simulink model "ssc_transformer"  (R2016b)
settings: Solver=VariableStepAuto  StartTime=0.0  StopTime=1  MaxStep=5e-5  RelTol=1e-3  EnableMultiTasking=on
PreLoadFcn:
  | L1 = 0.75*2.54e-2;  % 0.75 inch
  | L2 = 1.5*2.54e-2 ;  % 1.5 inch
  | Area = L1*L1;
libraries: fl_lib x19, nesl_utility x7
CloseFcn:
  | try,close(h1_ssc_transformer),end
  | clear h1_ssc_transformer
  | clear simlog_ssc_transformer
Description:
  | Electrical Transformer
  | 
  | Copyright 2008-2016 The MathWorks, Inc.
settings Model: Creator=MathWorks  LastModifiedBy=SHAAD
settings DataIOCC: LimitDataPoints=on  SaveFormat=Array
settings OptimizationCC: LifeSpan=inf
settings DebuggingCC: SolverPrmCheckMsg=warning  AllowSymbolicDim=off  SFUnexpectedBacktrackingDiag=warning  SFNoUnconditionalDefaultTransitionDiag=warning  SFExecutionAtInitializationDiag=none
settings HardwareCC: ProdBitPerPointer=32  ProdBitPerSizeT=32  ProdBitPerPtrDiffT=32  ProdLargestAtomicFloat=None  ProdIntDivRoundTo=Undefined  ProdEndianess=Unspecified  ProdWordSize=32  ProdHWDeviceType=32-bit Generic
settings ModelReferenceCC: PropagateSignalLabelsOutOfModel=off
settings GRTTargetCC: TargetLangStandard=C89/C90 (ANSI)  GeneratePreprocessorConditionals=Disable all
settings ConfigComp: CovMetricSettings=dw  CovHtmlReporting=on  CovSaveCumulativeToWorkspaceVar=on  CovSaveSingleToWorkspaceVar=on  CovExternalEMLEnable=off  CovSFcnEnable=off
settings SimscapeCC: SimscapeLogType=all  SimscapeLogSimulationStatistics=on  SimscapeLogName=simlog_ssc_transformer  SimscapeLogDataHistory=30000

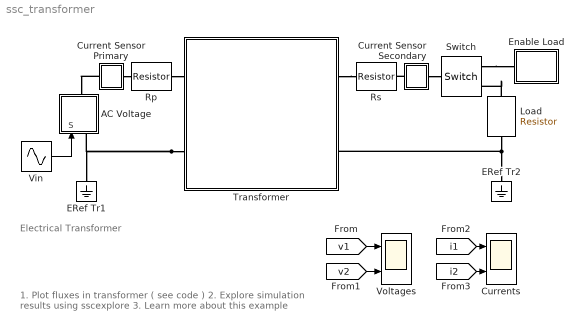
== system ssc_transformer ==
  note: 1. Plot fluxes in transformer ( see code )
      | 2. Explore simulation results using sscexplore
      | 3. Learn more about this example
  note: Electrical Transformer
  AC Voltage : Subsystem
  Current Sensor Primary : Subsystem
      mask Display: disp('vi1')
  Current Sensor Secondary : Subsystem
      mask Display: disp('vi2')
  Currents : Scope  NumInputPorts=2
  ERef Tr1 : fl_lib/Electrical/Electrical Elements/Electrical Reference
  ERef Tr2 : fl_lib/Electrical/Electrical Elements/Electrical Reference
  Enable Load : Subsystem
  Load : fl_lib/Electrical/Electrical Elements/Resistor  R=2.88 Ohm  i_specify=off  i_priority=High  i=0 A  v_specify=off  v_priority=High  v=0 V
  Rp : fl_lib/Electrical/Electrical Elements/Resistor  R=8.4683 Ohm  i_specify=off  i_priority=High  i=0 A  v_specify=off  v_priority=High  v=0 V
  Rs : fl_lib/Electrical/Electrical Elements/Resistor  R=8.4683/100 Ohm  i_specify=off  i_priority=High  i=0 A  v_specify=off  v_priority=High  v=0 V
  Switch : fl_lib/Electrical/Electrical Elements/Switch  R_closed=0.01 Ohm  G_open=1e-8 1/Ohm  Threshold=0  i_specify=off  i_priority=High  i=0 A  v_specify=off  v_priority=High  v=0 V
  Transformer : Subsystem  Tag=PublishSubsystem
      mask Display:
      | % Primary Coil
      | plot(cos(+pi/2:0.1:3*pi/2)*0.10-0.3,sin(+pi/2:0.1:3*pi/2)*0.10+0.4);
      | plot(cos(+pi/2:0.1:3*pi/2)*0.10-0.3,sin(+pi/2:0.1:3*pi/2)*0.10+0.2);
      | plot(cos(+pi/2:0.1:3*pi/2)*0.10-0.3,sin(+pi/2:0.1:3*pi/2)*0.10+0.0);
      | plot(cos(+pi/2:0.1:3*pi/2)*0.10-0.3,sin(+pi/2:0.1:3*pi/2)*0.10-0.2);
      | plot(cos(+pi/2:0.1:3*pi/2)*0.10-0.3,sin(+pi/2:0.1:3*pi/2)*0.10-0.4);
      | plot([-0.3 -0.3],[-0.6 -0.5]);plot([-0.3 -0.8],[-0.6 -0.6]);
      | plot([-0.3 -0.3],[+0.6 +0.5]);plot([-0.3 -0.8],[+0.6 +0.6]);
      | 
      | % Secondary Coil
      | plot(cos(-pi/2:0.1:pi/2)*0.10+0.3,sin(-pi/2:0.1:pi/2)*0.10+0.4);
      | plot(cos(-pi/2:0.1:pi/2)*0.10+0.3,sin(-pi/2:0.1:pi/2)*0.10+0.2);
      | plot(cos(-pi/2:0.1:pi/2)*0.10+0.3,sin(-pi/2:0.1:pi/2)*0.10+0.0);
      | plot(cos(-pi/2:0.1:pi/2)*0.10+0.3,sin(-pi/2:0.1:pi/2)*0.10-0.2);
      | plot(cos(-pi/2:0.1:pi/2)*0.10+0.3,sin(-pi/2:0.1:pi/2)*0.10-0.4);
      | plot([0.3 0.3],[-0.6 -0.5]);plot([0.3 0.8],[-0.6 -0.6]);
      | plot([0.3 0.3],[+0.6 +0.5]);plot([0.3 0.8],[+0.6 +0.6]);
      | 
      | % Plot points to set plot range
      | color('white');plot(1.1,1.1);plot(-1.1,-1.1)
      | color('black');
      | 
      | color('red')
      | port_label('LConn',1,'+1');
      | port_label('LConn',2,'-1');
      | port_label('RConn',1,'+2');
      | port_label('RConn',2,'-2');
      | color('black');
  Vin : Sin  Amplitude=120*sqrt(2)  Frequency=2*pi*60  Phase=pi/2  SampleTime=0
  Voltages : Scope  NumInputPorts=2
  wires:
  [v2] -> Voltages/2
  [v1] -> Voltages/1
  [i2] -> Currents/2
  [i1] -> Currents/1
  Vin/1 -> AC Voltage/1(S)
  connections:
  Current Sensor Secondary/RConn1 -- Switch/LConn1
  Load/RConn1 -- ERef Tr2/LConn1 -- Transformer/RConn2
  Load/LConn1 -- Switch/RConn2
  Rp/LConn1 -- Transformer/LConn1
  Transformer/RConn1 -- Rs/RConn1
  Current Sensor Secondary/LConn1 -- Rs/LConn1
  Transformer/LConn2 -- AC Voltage/LConn1 -- ERef Tr1/LConn1
  Current Sensor Primary/RConn1 -- Rp/RConn1
  Current Sensor Primary/LConn1 -- AC Voltage/RConn1
  Switch/RConn1 -- Enable Load/LConn1

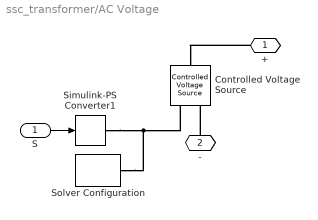
== system ssc_transformer/AC Voltage ==
  S : Inport
  Controlled Voltage Source : fl_lib/Electrical/Electrical Sources/Controlled Voltage Source
  Simulink-PS Converter1 : nesl_utility/Simulink-PS Converter  PhysicalDomain=network_engine_domain  SubClassName=ps_input  LeftPortType=input  RightPortType=output  PseudoPeriodic=off  Frequencies=[]  NoiseDistribution=none  NoiseParameters=[]  Unit=1  AffineConversion=off  InputFiltering=off  SimscapeFilterOrder=1  InputFilterTimeConstant=.001  UdotUserProvided=0
  Solver Configuration : nesl_utility/Solver Configuration  PhysicalDomain=network_engine_domain  SubClassName=solver  LeftPortType=input  RightPortType=generic  Accelerate=off  Tones=[]  Harmonics=[]  SimulateNoise=off  Profile=off  UseLocalSampling=off  EnableSwitchedLinearOptims=on  FrequencyDomain=off  UseCCode=off  RelTol=0.001  AbsTol=1e-06  MinStep=1e-09  ToWorkspace=off  RevertToSquareIcSolve=off  NumHomotopyIterations=100  PhasorMode=off  PhasorModeNumHarmonics=1  OverrideAbsTol=off  DoDC=off  ResidualTolerance=1e-9  UseLocalSolver=off  LocalSolverChoice=NE_BACKWARD_EULER_ADVANCER  LocalSolverSampleTime=.001  DoFixedCost=off  MaxNonlinIter=3  MaxModeIter=2  LinearAlgebra=Sparse  DelaysMemoryBudget=1024  AutomaticFiltering=on  FilteringTimeConstant=0.001
  + : PMIOPort  Port=1  Side=Right
  - : PMIOPort  Port=2  Side=Left
  wires:
  S/1 -> Simulink-PS Converter1/1
  connections:
  Simulink-PS Converter1/RConn1 -- Solver Configuration/RConn1 -- Controlled Voltage Source/RConn1
  +/RConn1 -- Controlled Voltage Source/LConn1
  -/RConn1 -- Controlled Voltage Source/RConn2

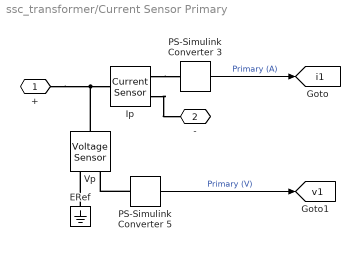
== system ssc_transformer/Current Sensor Primary ==
  ERef : fl_lib/Electrical/Electrical Elements/Electrical Reference
  Ip : fl_lib/Electrical/Electrical Sensors/Current Sensor
  PS-Simulink Converter 3 : nesl_utility/PS-Simulink Converter  PhysicalDomain=network_engine_domain  SubClassName=ps_output  LeftPortType=input  RightPortType=output  PseudoPeriodic=off  Frequencies=[]  Unit=1  AffineConversion=off
  PS-Simulink Converter 5 : nesl_utility/PS-Simulink Converter  PhysicalDomain=network_engine_domain  SubClassName=ps_output  LeftPortType=input  RightPortType=output  PseudoPeriodic=off  Frequencies=[]  Unit=1  AffineConversion=off
  Vp : fl_lib/Electrical/Electrical Sensors/Voltage Sensor
  + : PMIOPort  Port=1  Side=Left
  - : PMIOPort  Port=2  Side=Right
  tag scope: i1=global, v1=global
  wires:
  PS-Simulink Converter 3/1 -> [i1]  "Primary (A)"
  PS-Simulink Converter 5/1 -> [v1]  "Primary (V)"
  connections:
  Ip/RConn2 -- -/RConn1
  +/RConn1 -- Vp/LConn1 -- Ip/LConn1
  Ip/RConn1 -- PS-Simulink Converter 3/LConn1
  PS-Simulink Converter 5/LConn1 -- Vp/RConn1
  ERef/LConn1 -- Vp/RConn2

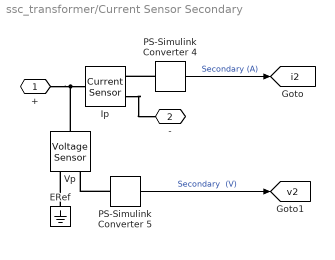
== system ssc_transformer/Current Sensor Secondary ==
  ERef : fl_lib/Electrical/Electrical Elements/Electrical Reference
  Ip : fl_lib/Electrical/Electrical Sensors/Current Sensor
  PS-Simulink Converter 4 : nesl_utility/PS-Simulink Converter  PhysicalDomain=network_engine_domain  SubClassName=ps_output  LeftPortType=input  RightPortType=output  PseudoPeriodic=off  Frequencies=[]  Unit=1  AffineConversion=off
  PS-Simulink Converter 5 : nesl_utility/PS-Simulink Converter  PhysicalDomain=network_engine_domain  SubClassName=ps_output  LeftPortType=input  RightPortType=output  PseudoPeriodic=off  Frequencies=[]  Unit=1  AffineConversion=off
  Vp : fl_lib/Electrical/Electrical Sensors/Voltage Sensor
  + : PMIOPort  Port=1  Side=Left
  - : PMIOPort  Port=2  Side=Right
  tag scope: i2=global, v2=global
  wires:
  PS-Simulink Converter 4/1 -> [i2]  "Secondary (A)"
  PS-Simulink Converter 5/1 -> [v2]  "Secondary  (V)"
  connections:
  PS-Simulink Converter 4/LConn1 -- Ip/RConn1
  +/RConn1 -- Vp/LConn1 -- Ip/LConn1
  Ip/RConn2 -- -/RConn1
  PS-Simulink Converter 5/LConn1 -- Vp/RConn1
  ERef/LConn1 -- Vp/RConn2

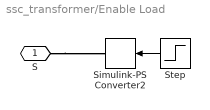
== system ssc_transformer/Enable Load ==
  Simulink-PS Converter2 : nesl_utility/Simulink-PS Converter  PhysicalDomain=network_engine_domain  SubClassName=ps_input  LeftPortType=input  RightPortType=output  PseudoPeriodic=off  Frequencies=[]  NoiseDistribution=none  NoiseParameters=[]  Unit=1  AffineConversion=off  InputFiltering=off  SimscapeFilterOrder=1  InputFilterTimeConstant=.001  UdotUserProvided=0
  Step : Step  Time=0.5  SampleTime=0
  S : PMIOPort  Port=1  Side=Left
  wires:
  Step/1 -> Simulink-PS Converter2/1
  connections:
  S/RConn1 -- Simulink-PS Converter2/RConn1

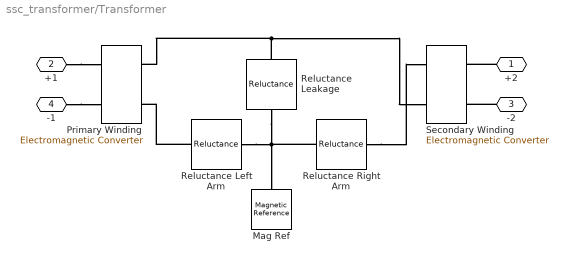
== system ssc_transformer/Transformer ==
  Mag Ref : fl_lib/Magnetic/Magnetic Elements/Magnetic Reference
  Primary Winding : fl_lib/Magnetic/Magnetic Elements/Electromagnetic Converter  Nw=1200  i_specify=off  i_priority=High  i=0 A  v_specify=off  v_priority=High  v=0 V  mmf_specify=off  mmf_priority=High  mmf=0 A  phi_specify=off  phi_priority=High  phi=0 Wb
  Reluctance Leakage : fl_lib/Magnetic/Magnetic Elements/Reluctance  g=L2 m  CSA=Area m^2  mur=1  phi_specify=off  phi_priority=High  phi=0 Wb  mmf_specify=off  mmf_priority=High  mmf=0 A
  Reluctance Left Arm : fl_lib/Magnetic/Magnetic Elements/Reluctance  g=2*(L1+L2) m  CSA=Area m^2  mur=25706  phi_specify=off  phi_priority=High  phi=0 Wb  mmf_specify=off  mmf_priority=High  mmf=0 A
  Reluctance Right Arm : fl_lib/Magnetic/Magnetic Elements/Reluctance  g=2*(L1+L2) m  CSA=Area m^2  mur=25706  phi_specify=off  phi_priority=High  phi=0 Wb  mmf_specify=off  mmf_priority=High  mmf=0 A
  Secondary Winding : fl_lib/Magnetic/Magnetic Elements/Electromagnetic Converter  Nw=120  i_specify=off  i_priority=High  i=0 A  v_specify=off  v_priority=High  v=0 V  mmf_specify=off  mmf_priority=High  mmf=0 A  phi_specify=off  phi_priority=High  phi=0 Wb
  +2 : PMIOPort  Port=1  Side=Right
  +1 : PMIOPort  Port=2  Side=Left
  -2 : PMIOPort  Port=3  Side=Right
  -1 : PMIOPort  Port=4  Side=Left
  connections:
  +2/RConn1 -- Secondary Winding/LConn1
  +1/RConn1 -- Primary Winding/LConn1
  -2/RConn1 -- Secondary Winding/LConn2
  -1/RConn1 -- Primary Winding/LConn2
  Reluctance Left Arm/LConn1 -- Primary Winding/RConn2
  Reluctance Leakage/LConn1 -- Secondary Winding/RConn2 -- Primary Winding/RConn1
  Reluctance Right Arm/LConn1 -- Mag Ref/LConn1 -- Reluctance Leakage/RConn1 -- Reluctance Left Arm/RConn1
  Reluctance Right Arm/RConn1 -- Secondary Winding/RConn1
